simulink model "mono_radiomodel"  (R2020a)
settings: Solver=FixedStepDiscrete  StartTime=0.0  StopTime=10  RelTol=1e-3  EnableMultiTasking=on
libraries: dspsigops x4, dspsnks4 x1, dspvision x1
Description:
  | This model uses the Digital Up-Converter (DUC) and Digital Down-Converter (DDC) blocks to create a Family Radio Service (FRS) transmitter and receiver.
settings Model: Creator=The MathWorks, Inc.  LastModifiedBy=agopiset
settings DataIOCC: LimitDataPoints=on  SaveFormat=Array  SaveOutput=off  SignalLogging=off  DSMLogging=off  SaveTime=off  ReturnWorkspaceOutputs=off
settings OptimizationCC: DefaultParameterBehavior=Inlined  EnhancedBackFolding=on  PassReuseOutputArgsAs=Individual arguments  SimCompilerOptimization=on  OptimizeBlockOrder=speed  DifferentSizesBufferReuse=on  OptimizationCustomize=off  EfficientTunableParamExpr=on
settings DebuggingCC: SolverPrmCheckMsg=warning  ParameterTunabilityLossMsg=error  AllowSymbolicDim=off  SFUnexpectedBacktrackingDiag=warning  SFNoUnconditionalDefaultTransitionDiag=warning  SFExecutionAtInitializationDiag=none  ArithmeticOperatorsInVariantConditions=warning
settings HardwareCC: ProdBitPerPointer=32  ProdBitPerSizeT=32  ProdBitPerPtrDiffT=32  ProdLargestAtomicFloat=None  ProdIntDivRoundTo=Undefined  ProdEndianess=Unspecified  ProdWordSize=32  ProdHWDeviceType=32-bit Generic
settings ModelReferenceCC: PropagateSignalLabelsOutOfModel=off
settings SFSimCC: SimUseLocalCustomCode=off  MATLABDynamicMemAlloc=off  CustomCodeUndefinedFunction=UseInterfaceOnly
settings RTWCC: SystemTargetFile=ert.tlc  TemplateMakefile=ert_default_tmf  GenerateReport=on  RTWUseLocalCustomCode=off  IncludeHyperlinkInReport=on  LaunchReport=on  GenerateTraceInfo=on  GenerateTraceReport=on  GenerateTraceReportSl=on  GenerateTraceReportSf=on  GenerateTraceReportEml=on
settings CodeAppCC: ForceParamTrailComments=on  IgnoreCustomStorageClasses=off  OperatorAnnotations=on  SimulinkDataObjDesc=on  SFDataObjDesc=on  InsertBlockDesc=on
settings ERTTargetCC: GenerateSampleERTMain=on  InlinedParameterPlacement=NonHierarchical  TargetOS=NativeThreadsExample  ERTCustomFileTemplate=example_file_process.tlc
settings ConfigComp: CovMetricSettings=dw  CovHtmlReporting=on  CovSaveCumulativeToWorkspaceVar=on  CovSaveSingleToWorkspaceVar=on  CovExternalEMLEnable=off  CovSFcnEnable=off

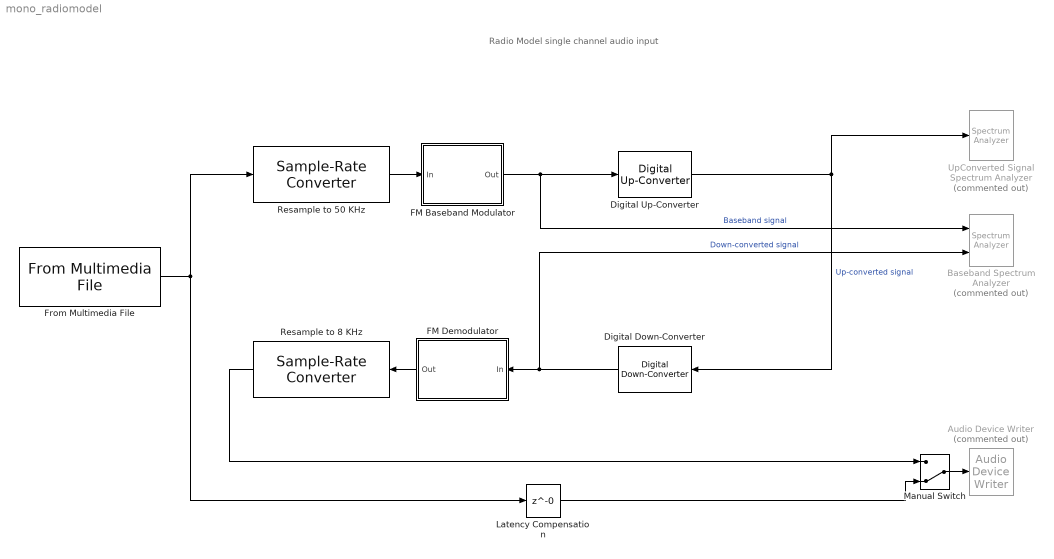
== system mono_radiomodel ==
  note: Radio Model
      | single channel audio input
  Audio Device Writer : dspsnks4/Audio Device Writer  Commented=on  Driver=DirectSound  Device=Default  InheritSampleRate=on  SampleRate=44100  BitDepth=16-bit integer  BufferSize=4096  NumBuffers=10  DefaultOutputChannelMapping=on  OutputChannelMapping=1:2  OutputNumUnderrunSamples=off  DriverIdx=1  DeviceWarnFlag=''
  Baseband Spectrum Analyzer : SpectrumAnalyzer  Commented=on  NumInputPorts=2
  Digital Down-Converter : dspsigops/Digital Down-Converter  DecimationFactor=40  MinimumOrderDesign=on  NumCICSections=3  SecondFilterOrder=12  ThirdFilterOrder=10  Bandwidth=12.5e3  StopbandFrequencySource=Property  StopbandFrequency=18.75e3  PassbandRipple=0.05  StopbandAttenuation=60  Oscillator=Sine wave  CenterFrequency=455e3  NumAccumulatorBits=16  NumQuantizedAccumulatorBits=12  Dither=on  NumDitherBits=4  InheritSampleRate=on  SampleRate=30000000  SimulateUsing=Code generation  outputMin=[]  outputMax=[]
      settings: SourceProductBaseCode=DS
  Digital Up-Converter : dspsigops/Digital Up-Converter  InterpolationFactor=40  MinimumOrderDesign=on  FirstFilterOrder=10  SecondFilterOrder=12  NumCICSections=3  Bandwidth=12.5e3  StopbandFrequencySource=Property  StopbandFrequency=18.75e3  PassbandRipple=0.05  StopbandAttenuation=60  Oscillator=Sine wave  CenterFrequency=455e3  NumAccumulatorBits=16  NumQuantizedAccumulatorBits=12  Dither=on  NumDitherBits=4  InheritSampleRate=on  SampleRate=300000  SimulateUsing=Code generation  outputMin=[]  outputMax=[]
      settings: SourceProductBaseCode=DS
  FM Baseband Modulator : Subsystem
  FM Demodulator : Subsystem
  From Multimedia File : dspvision/From Multimedia File  inputFilename=speech_dft_8kHz.wav  readRange=[1 Inf]  loop=on  numPlays=inf  outputStreams=Audio only  videoDataType=single  audioDataType=double  inheritSampleTime=on  userDefinedSampleTime=1/30  noAudioOutput=off  isIntensityVideo=off  fourcc=RGB  colorVideoFormat=Separate color signals  outputEOF=off  dataOrg=Column-major  audioFrameSize=1000  computeAudioFrameSize=off  outSamplingMode=Sample based  mask(From Multimedia File){}
      mask Display:
      | % This is a new mask on top of the base mask.
      | % Use "View base mask" link below to see the base mask.
      | fprintf("Audio .wav file\n8kHz, mono");
  Latency Compensation : Delay  DelayLength=0  InputProcessing=Columns as channels (frame based)
  Manual Switch : ManualSwitch  CurrentSetting=0
  Resample to 50 KHz : dspsigops/Sample-Rate Converter  InputSampleRate=8e3  OutputSampleRate=50e3  OutputRateTolerance=0  Bandwidth=6.25e3  StopbandAttenuation=80  SimulateUsing=Code generation
      settings: SourceProductBaseCode=DS
  Resample to 8 KHz : dspsigops/Sample-Rate Converter  InputSampleRate=50e3  OutputSampleRate=8e3  OutputRateTolerance=0  Bandwidth=6.25e3  StopbandAttenuation=80  SimulateUsing=Code generation
      settings: SourceProductBaseCode=DS
  UpConverted Signal Spectrum Analyzer : SpectrumAnalyzer  Commented=on
  wires:
  Manual Switch/1 -> Audio Device Writer/1
  Resample to 8 KHz/1 -> Manual Switch/1
  Latency Compensation/1 -> Manual Switch/2
  Resample to 50 KHz/1 -> FM Baseband Modulator/1(In)
  Digital Down-Converter/1 -> Baseband Spectrum Analyzer/2, FM Demodulator/1(In)  "Down-converted signal"
  FM Baseband Modulator/1(Out) -> Baseband Spectrum Analyzer/1, Digital Up-Converter/1  "Baseband signal"
  Digital Up-Converter/1 -> UpConverted Signal Spectrum Analyzer/1, Digital Down-Converter/1  "Up-converted signal"
  FM Demodulator/1(Out) -> Resample to 8 KHz/1
  From Multimedia File/1 -> Resample to 50 KHz/1, Latency Compensation/1

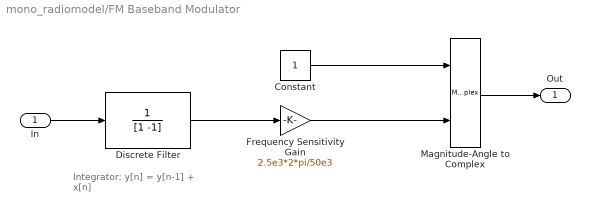
== system mono_radiomodel/FM Baseband Modulator ==
  note: Integrator:
      | y[n] = y[n-1] + x[n]
  In : Inport
  Constant : Constant  SampleTime=-1
  Discrete Filter : DiscreteFilter  Numerator=1  Denominator=[1 -1]  InputProcessing=Columns as channels (frame based)  FilterStructure=Direct form II transposed  a0EqualsOne=on
  Frequency Sensitivity Gain : Gain  Gain=2.5e3*2*pi/50e3
  Magnitude-Angle to Complex : MagnitudeAngleToComplex
  Out : Outport  VectorParamsAs1DForOutWhenUnconnected=off
  wires:
  Frequency Sensitivity Gain/1 -> Magnitude-Angle to Complex/2
  Discrete Filter/1 -> Frequency Sensitivity Gain/1
  In/1 -> Discrete Filter/1
  Magnitude-Angle to Complex/1 -> Out/1
  Constant/1 -> Magnitude-Angle to Complex/1

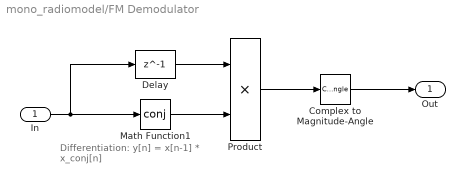
== system mono_radiomodel/FM Demodulator ==
  note: Differentiation:
      | y[n] = x[n-1] * x_conj[n]
  In : Inport
  Complex to Magnitude-Angle : ComplexToMagnitudeAngle  Output=Angle
  Delay : Delay  DelayLength=1  InitialCondition=0  InputProcessing=Columns as channels (frame based)
  Math Function1 : Math  Operator=conj  SignedPower=on  SaturateOnIntegerOverflow=on
  Product : Product  RndMeth=Zero
  Out : Outport  VectorParamsAs1DForOutWhenUnconnected=off
  wires:
  Complex to Magnitude-Angle/1 -> Out/1
  Math Function1/1 -> Product/2
  In/1 -> Math Function1/1, Delay/1
  Delay/1 -> Product/1
  Product/1 -> Complex to Magnitude-Angle/1
